simulink model "simpleIO_task"  (Simulink 3.00)
settings: Solver=ode45  SolverMode=SingleTasking  StartTime=0.0  StopTime=10.0  RelTol=1e-3
libraries: mathlib x5, inoutlib x2, genlib x1, arclib x1
settings Model: ExtModeTrigMode=normal  ExtModeArmWhenConnect=on  LastModifiedBy=mertlj

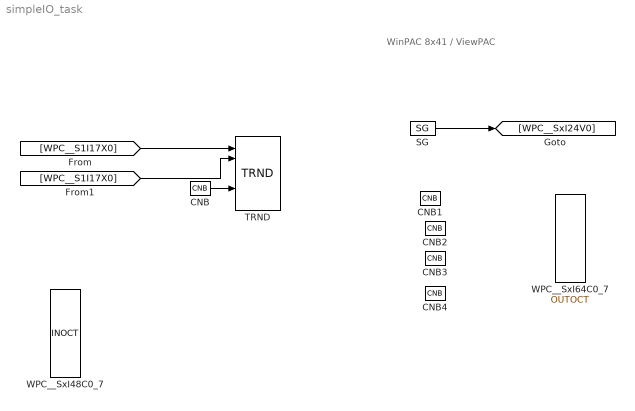
== system simpleIO_task ==
  note: WinPAC 8x41 / ViewPAC
  CNB : mathlib/CNB  YCN=on
  CNB1 : mathlib/CNB  YCN=on
  CNB2 : mathlib/CNB  YCN=off
  CNB3 : mathlib/CNB  YCN=on
  CNB4 : mathlib/CNB  YCN=off
  SG : genlib/SG  isig=1: SINE  amp=7.5  freq=0.1  phase=0  ifrunit=1: Hz  iphunit=1: degrees
  TRND : arclib/TRND  n=4  l=1000  btype=8: Double  ptype1=1: Store  ptype2=1: Store  ptype3=1: Store  ptype4=1: Store  pfac=1  afac=0  arc=0  id=1  Title=Trend Title
  WPC__SxI48C0_7 : inoutlib/INOCT
  WPC__SxI64C0_7 : inoutlib/OUTOCT
  wires:
  CNB/1 -> TRND/5
  [WPC__S1I17X0] -> TRND/1
  [WPC__S1I17X0] -> TRND/2
  SG/1 -> [WPC__SxI24V0]
